simulink model "IEEE80211a"  (Simulink 10.0)
settings: Solver=VariableStepDiscrete  StartTime=0.0  StopTime=inf  RelTol=1e-3  EnableMultiTasking=on
PreLoadFcn:
  | load IEEE80211a_init;
undefined symbols (not defined in the file): hyst, j, magnitude, params, QAM, thres
libraries: simulink x27, IEEE80211a_lib x19, dspsigops x19, dspmtrx3 x19, dspsigattribs x15, dspmlti3 x10, dspstat3 x6, dspmathops x5, dspindex x3, dspsrcs4 x3, dspbuff3 x2, dspxfrm3 x2
(part 1 of 2)
CloseFcn:
  | IEEE80211a_open_graphics('IEEE80211a/MATLAB graphics', 1)
settings Model: Creator=Martin Clark  LastModifiedBy=bhisma
settings DataIOCC: LimitDataPoints=on  SignalLoggingSaveFormat=ModelDataLogs  SaveOutput=off  SaveTime=off  SignalLoggingName=sigsOut
settings OptimizationCC: LifeSpan=auto
settings DebuggingCC: SaveWithParameterizedLinksMsg=none  SignalResolutionControl=TryResolveAllWithWarning  MultiTaskDSMMsg=warning  MultiTaskCondExecSysMsg=none  SFUnexpectedBacktrackingDiag=error  SFNoUnconditionalDefaultTransitionDiag=error  SFExecutionAtInitializationDiag=warning  ArithmeticOperatorsInVariantConditions=error
settings HardwareCC: TargetUnknown=on
settings SFSimCC: SimUseLocalCustomCode=on  SimParseCustomCode=off  CustomCodeUndefinedFunction=FilterOut
settings RTWCC: RTWUseLocalCustomCode=on
settings CodeAppCC: StateflowObjectComments=off
settings GRTTargetCC: TargetLangStandard=C99 (ISO)

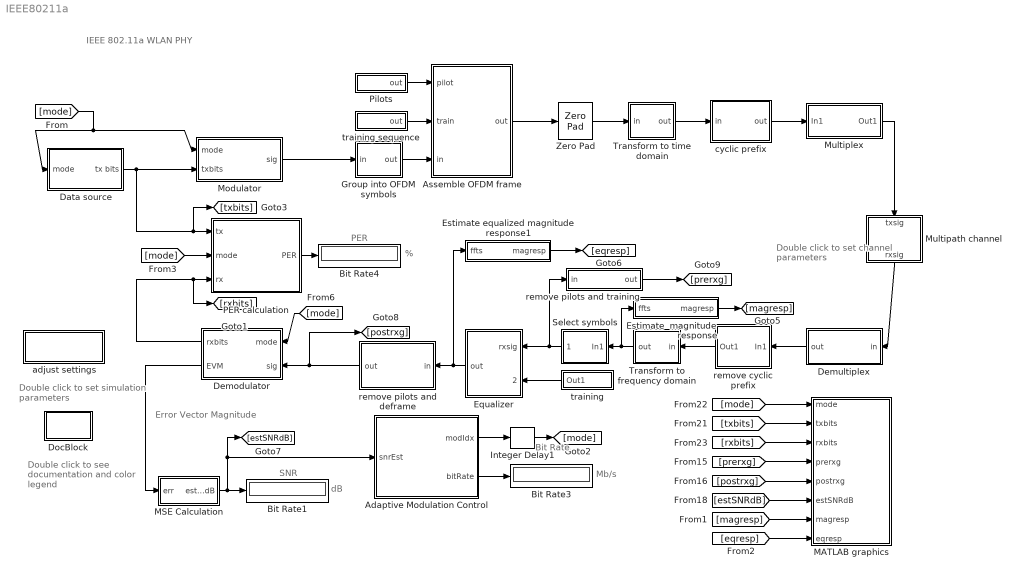
== system IEEE80211a ==
  note: IEEE 802.11a WLAN PHY
  note: Mb/s
  note: %
  note: Bit Rate
  note: Error Vector
      | Magnitude
  note: SNR
  note: dB
  note: Double click to set
      | channel parameters
  note: PER
  note: Double click to see
      |  documentation
      | and color legend
  note: Double click to set
      |  simulation parameters
  Adaptive Modulation Control : Stateflow chart  TreatAsAtomicUnit=on
  Assemble OFDM frame : Subsystem
      mask Display: disp('Assemble\nOFDM Frames')
  Bit Rate1 : Display
  Bit Rate3 : Display
  Bit Rate4 : Display
  Data source : Subsystem
      mask Display: disp('Variable-Rate\nData source')
  Demodulator : Subsystem  mask(IEEE 802.11a demodulator-decoder bank.){nSymbolsPerFrame=params.numTxSymbols, vtbd_set=params.vtbd_set}
      mask prompts: nSymbolsPerFrame "Number of symbols per frame:"; vtbd_set "vtbd set"
      mask init:
      | numModulators = 8;
      | modulation = {'BPSK' 'BPSK' 'QPSK' 'QPSK' '16-QAM' '16-QAM' '64-QAM' '64-QAM'};
      | code = {'1/2' '3/4' '1/2' '3/4' '1/2' '3/4' '2/3' '3/4'};
      | 
      | % modulation-specific
      | TS1 = 'poly2trellis(7, [171 133])';
      | TS2 = 'poly2trellis(7, [133 171])';
      | trellisStructure = {TS1 TS1 TS1 TS1 TS1 TS1 TS2 TS2};
      | 
      | % code-specific
      | PV = {'[1]', '[1 1 1 0].''', '[1 1 1 0 0 1].''', '[1]'};
      | punctureVector = {PV{1} PV{3} PV{1} PV{3} PV{1} PV{3} PV{2} PV{3}};
      | 
      | for n = 1:numModulators
      |     blk = [gcb '/Demodulator ' num2str(n)];
      |     set_param(blk, 'numSymbols', num2str(nSymbolsPerFrame));
      |     set_param(blk, 'modulation', modulation{n});
      |     set_param(blk, 'code', code{n});
      |     set_param(blk, 'trellisStructure', trellisStructure{n});
      |     set_param(blk, 'punctureVector', punctureVector{n});
      | end
      mask Display: disp('Demodulator\nBank')
  Demultiplex : Subsystem
      mask Display: disp('Demultiplex\nOFDM Frames')
  DocBlock : Subsystem  mask(DocBlock){ECoderFlag=, DocumentType=Text}
      mask prompts: ECoderFlag "E Coder Flag"; DocumentType "Document Type"
      mask help: Use this block to save long descriptive text with the model. Double-clicking the block will open an editor.
      settings: CopyFcn=docblock('breaklink',gcb);  DeleteFcn=docblock('close_document',gcb);  PreSaveFcn=docblock('save_document',gcb);  OpenFcn=docblock('edit_document',gcb);
      mask TypeOptions DocumentType: Text | RTF | HTML
      mask Display:
      | plot([.8 0 0 1 1 .8 .8 1],[1 1 0 0 .8 1 .8 .8]);
      | text(.5,.5,'DOC','horizontalalignment','center');
  Equalizer : Subsystem
      mask Display: disp('Frequency\nDomain\nEqualizer')
  Estimate  magnitude response : Subsystem
      mask Display: disp('Power Spectrum')
  Estimate equalized magnitude response1 : Subsystem
      mask Display: disp('Power Spectrum')
  Group into OFDM symbols : Subsystem
      mask Display: disp('OFDM\nSymbols')
  Integer Delay1 : dspsigops/Integer Delay  delay=1  ic=1  reset_popup=None
      settings: AttributesFormatString=\n  SourceProductName=DSP System Toolbox  SourceProductBaseCode=DS
  MATLAB graphics : Subsystem  mask(User-defined graphics.){graphicsName=IEEE80211a_graphics, portNames={'mode', 'txbits', 'rxbits', 'avSNRdB', 'prerxg', 'postrxg', 'estSNRdB', 'magresp', 'eqresp'}, convertMode=structure, extraParams=params}
      mask prompts: graphicsName "Graphics filename (without .fig or .m extension):"; portNames "Port names (cell array):"; convertMode "Data conversion mode:"; extraParams "Additional parameters:"
      mask init:
      | % derive input_names
      | bl = length(gcb);
      | long_names = find_system(gcb,...
      |     'lookundermasks','All',...
      |     'searchdepth', 1,...
      |     'BlockType','Inport');
      | lln = length(long_names);
      | input_names = cell(1, lln);
      | for i=1:lln
      | 	input_names{i}=long_names{i}(bl+2 : end);
      | end
      | 
      | if strcmp(get_param(gcb, 'LinkStatus'), 'resolved')
      | 	set_param(gcb, 'LinkStatus', 'inactive');
      | end
      settings: OpenFcn=IEEE80211a_open_graphics(gcb, 0);
      mask TypeOptions convertMode: cell array | structure
      mask Display: disp('Signal\nVisualization\n\nDouble click to\nopen/close')
  MSE Calculation : Subsystem
      mask Display: disp('SNR\nEstimation')
  Modulator : Subsystem  mask(IEEE 802.11a modulator-coder bank.){nSymbolsPerFrame=params.numTxSymbols}
      mask prompts: nSymbolsPerFrame "Number of symbols per frame:"
      mask init:
      | numModulators = 8;
      | modulation = {'BPSK' 'BPSK' 'QPSK' 'QPSK' '16-QAM' '16-QAM' '64-QAM' '64-QAM'};
      | code = {'1/2' '3/4' '1/2' '3/4' '1/2' '3/4' '2/3' '3/4'};
      | 
      | % modulation-specific
      | TS1 = 'poly2trellis(7, [171 133])';
      | TS2 = 'poly2trellis(7, [133 171])';
      | trellisStructure = {TS1 TS1 TS1 TS1 TS1 TS1 TS2 TS2};
      | 
      | % code-specific
      | PV = {'[1]', '[1 1 1 0].''', '[1 1 1 0 0 1].''', '[1]'};
      | punctureVector = {PV{1} PV{3} PV{1} PV{3} PV{1} PV{3} PV{2} PV{3}};
      | 
      | for n = 1:numModulators
      |     blk = [gcb '/Modulator ' num2str(n)];
      |     set_param(blk, 'numSymbols', num2str(nSymbolsPerFrame));
      |     set_param(blk, 'modulation', modulation{n});
      |     set_param(blk, 'code', code{n});
      |     set_param(blk, 'trellisStructure', trellisStructure{n});
      |     set_param(blk, 'punctureVector', punctureVector{n});
      | end
      mask Display: disp('Modulator\nBank')
  Multipath channel : Subsystem  mask(Multipath channel model parameters.){fadingMode=Dispersive fading, maxDoppler=200, SNRdB=30, chanSamplePeriod=params.chanSamplePeriod}
      mask prompts: fadingMode "Fading mode:"; maxDoppler "Maximum Doppler shift (Hz):"; SNRdB "SNR (dB):"; chanSamplePeriod "Channel sample period (s):"
      mask TypeOptions fadingMode: No fading | Flat fading | Dispersive fading
      mask Display: disp('Multipath\nChannel')
  Multiplex : Subsystem
      mask Display: disp('Multiplex\nOFDM Frames')
  PER calculation : Subsystem
      mask Display: disp('Packet Error Rate\nCalculation')
  Pilots : Subsystem
      mask Display: disp('Pilots')
  Select symbols : Subsystem
      mask Display: disp('Remove\nZeros')
  Transform to frequency domain : Subsystem
      mask Display: disp('FFT')
  Transform to time domain : Subsystem
      mask Display: disp('IFFT')
  Zero Pad : dspsigops/Zero Pad  padSigAt=End  zpadAlong=Columns  padNumOutRowsSpecMethod=User-specified  numOutRows=params.NFFT  padNumOutColsSpecMethod=User-specified  numOutCols=1  trunc_flag=None
      settings: SourceProductName=DSP System Toolbox  SourceProductBaseCode=DS
  adjust settings : Subsystem  Priority=1  mask(IEEE 802.11a model - Settings.){symbol_period=0.08e-6, OFDMSymPerFrame=20, OFDMTrainPerFrame=4, SNR0_dB=[10 11 14 18 22 26 28], hyst=3, vtbd=34}
      mask prompts: symbol_period "Symbol period (seconds):"; OFDMSymPerFrame "Number of OFDM symbols per transmit block:"; OFDMTrainPerFrame "Number of OFDM symbols in training sequence:"; SNR0_dB "Low-SNR thresholds (dB) -- no threshold for lowest modulation:"; hyst "Hysteresis factor for adaptive modulation (dB):"; vtbd "Viterbi traceback depth:"
      mask help: Parameter settings for IEEE 802.11a model.
      mask init:
      | params = IEEE80211a_settings(...
      | 	symbol_period, ...
      | 	OFDMSymPerFrame, ...
      | 	OFDMTrainPerFrame, ...
      | 	vtbd);
      | 
      | assignin('base', 'params', params);
      | assignin('base', 'thres', SNR0_dB);
      | assignin('base', 'hyst', hyst);
      mask Help: Parameter settings for IEEE 802.11a model.
      mask Display: disp('Simulation\nSettings')
  cyclic prefix : Subsystem
      mask Display: disp('Append\nCyclic\nPrefix')
  remove cyclic prefix : Subsystem
      mask Display: disp('Remove\nCyclic\nPrefix')
  remove pilots and deframe : Subsystem
      mask Display: disp('Disassemble\nOFDM Frames')
  remove pilots and training : Subsystem
      mask Display: disp('Constellation')
  training : Subsystem
      mask Display: disp('Training')
  training sequence : Subsystem
      mask Display: disp('Training')
  wires:
  cyclic prefix/1(out) -> Multiplex/1(In1)
  [mode] -> Demodulator/1(mode)
  Modulator/1(sig) -> Group into OFDM symbols/1(in)
  Demodulator/2(EVM) -> MSE Calculation/1(err)
  Data source/1(tx bits) -> Modulator/2(txbits), PER calculation/1(tx), [txbits]
  PER calculation/1(PER) -> Bit Rate4/1
  Demodulator/1(rxbits) -> PER calculation/3(rx), [rxbits]
  Integer Delay1/1 -> [mode]
  Adaptive Modulation Control/2(bitRate) -> Bit Rate3/1
  Adaptive Modulation Control/1(modIdx) -> Integer Delay1/1
  Transform to time domain/1(out) -> cyclic prefix/1(in)
  Assemble OFDM frame/1(out) -> Zero Pad/1
  training sequence/1(out) -> Assemble OFDM frame/2(train)
  Pilots/1(out) -> Assemble OFDM frame/1(pilot)
  Estimate  magnitude response/1(magresp) -> [magresp]
  Estimate equalized magnitude response1/1(magresp) -> [eqresp]
  Multipath channel/1(rxsig) -> Demultiplex/1(in)
  remove cyclic prefix/1(Out1) -> Transform to frequency domain/1(in)
  Equalizer/1(out) -> remove pilots and deframe/1(in), Estimate equalized magnitude response1/1(ffts)
  remove pilots and deframe/1(out) -> [postrxg], Demodulator/2(sig)
  training/1(Out1) -> Equalizer/2(trainsig)
  Transform to frequency domain/1(out) -> Estimate  magnitude response/1(ffts), Select symbols/1(In1)
  Group into OFDM symbols/1(out) -> Assemble OFDM frame/3(in)
  Multiplex/1(Out1) -> Multipath channel/1(txsig)
  Demultiplex/1(out) -> remove cyclic prefix/1(In1)
  [mode] -> Data source/1(mode), Modulator/1(mode)
  Zero Pad/1 -> Transform to time domain/1(in)
  remove pilots and training/1(out) -> [prerxg]
  Select symbols/1(Out1) -> Equalizer/1(rxsig), remove pilots and training/1(in)
  MSE Calculation/1(estSNRdB) -> Bit Rate1/1, Adaptive Modulation Control/1(snrEst), [estSNRdB]
  [mode] -> MATLAB graphics/1(mode)
  [txbits] -> MATLAB graphics/2(txbits)
  [rxbits] -> MATLAB graphics/3(rxbits)
  [prerxg] -> MATLAB graphics/4(prerxg)
  [postrxg] -> MATLAB graphics/5(postrxg)
  [estSNRdB] -> MATLAB graphics/6(estSNRdB)
  [magresp] -> MATLAB graphics/7(magresp)
  [eqresp] -> MATLAB graphics/8(eqresp)
  [mode] -> PER calculation/2(mode)

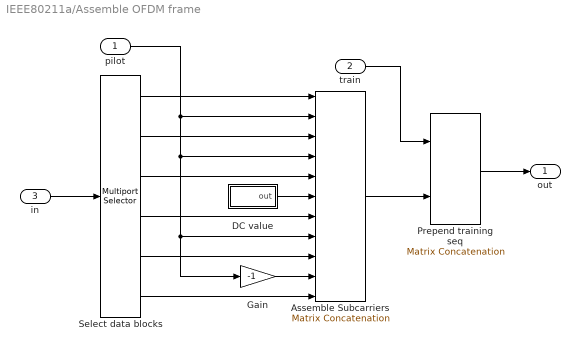
== system IEEE80211a/Assemble OFDM frame ==
  pilot : Inport
  train : Inport  Port=2
  in : Inport  Port=3
  Assemble Subcarriers : simulink/Math Operations/Matrix Concatenation  numInports=11  catMethod=Vertical
      settings: SourceProductName=Simulink  SourceProductBaseCode=SL
  DC value : Subsystem
      mask Display: disp('Zero DC')
  Gain : Gain  Gain=-1  SaturateOnIntegerOverflow=on  OutDataTypeStr=Inherit: Same as input  ParamDataTypeStr=Inherit: Same as input
  Prepend training seq : simulink/Math Operations/Matrix Concatenation  numInports=2  catMethod=Horizontal
      settings: SourceProductName=Simulink  SourceProductBaseCode=SL
  Select data blocks : dspindex/Multiport Selector  rowsOrCols=Rows  idxCellArray={1:5, 6:18, 19:24, 25:30, 31:43, 44:48}  idxErrMode=Clip Index
  out : Outport
  wires:
  Select data blocks/1 -> Assemble Subcarriers/1
  Select data blocks/2 -> Assemble Subcarriers/3
  Select data blocks/3 -> Assemble Subcarriers/5
  Select data blocks/4 -> Assemble Subcarriers/7
  Select data blocks/5 -> Assemble Subcarriers/9
  Select data blocks/6 -> Assemble Subcarriers/11
  Gain/1 -> Assemble Subcarriers/10
  pilot/1 -> Gain/1, Assemble Subcarriers/8, Assemble Subcarriers/4, Assemble Subcarriers/2
  Assemble Subcarriers/1 -> Prepend training seq/2
  train/1 -> Prepend training seq/1
  Prepend training seq/1 -> out/1
  DC value/1(out) -> Assemble Subcarriers/6
  in/1 -> Select data blocks/1

== system IEEE80211a/Data source ==
  mode : Inport
  Binary source : Subsystem  TreatAsAtomicUnit=on  mask{sample_time=params.minBitPeriod, samp_per_frame=params.nSource}
      mask prompts: sample_time "Sample time:"; samp_per_frame "Samples per frame:"
      mask help: Enabled binary data source
  Buffer : dspbuff3/Buffer  N=params.maxBitsPerBlock  V=0  ic=0
      settings: SourceProductName=DSP System Toolbox  SourceProductBaseCode=DS
  Source enable : Subsystem
  tx bits : Outport
  wires:
  Binary source/1(data out) -> Buffer/1
  Buffer/1 -> tx bits/1
  mode/1 -> Source enable/1(mode)
  Source enable/1(enable) -> Binary source/Enable

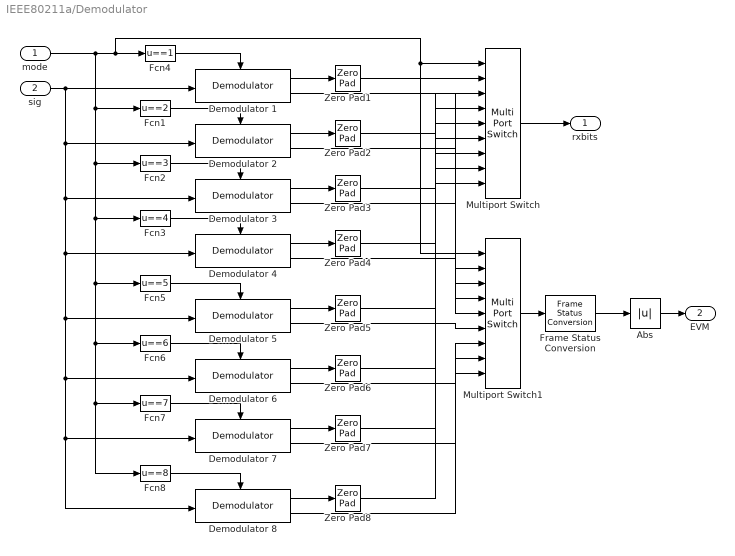
== system IEEE80211a/Demodulator ==
  mode : Inport
  sig : Inport  Port=2
  Abs : Abs  SaturateOnIntegerOverflow=on
  Demodulator 1 : IEEE80211a_lib/Demodulator  numSymbols=960  modulation=BPSK  code=1/2  trellisStructure=poly2trellis(7, [171 133])  punctureVector=[1]  vtbd=34
  Demodulator 2 : IEEE80211a_lib/Demodulator  numSymbols=960  modulation=BPSK  code=3/4  trellisStructure=poly2trellis(7, [171 133])  punctureVector=[1 1 1 0 0 1].'  vtbd=34
  Demodulator 3 : IEEE80211a_lib/Demodulator  numSymbols=960  modulation=QPSK  code=1/2  trellisStructure=poly2trellis(7, [171 133])  punctureVector=[1]  vtbd=34
  Demodulator 4 : IEEE80211a_lib/Demodulator  numSymbols=960  modulation=QPSK  code=3/4  trellisStructure=poly2trellis(7, [171 133])  punctureVector=[1 1 1 0 0 1].'  vtbd=34
  Demodulator 5 : IEEE80211a_lib/Demodulator  numSymbols=960  modulation=16-QAM  code=1/2  trellisStructure=poly2trellis(7, [171 133])  punctureVector=[1]  vtbd=34
  Demodulator 6 : IEEE80211a_lib/Demodulator  numSymbols=960  modulation=16-QAM  code=3/4  trellisStructure=poly2trellis(7, [171 133])  punctureVector=[1 1 1 0 0 1].'  vtbd=34
  Demodulator 7 : IEEE80211a_lib/Demodulator  numSymbols=960  modulation=64-QAM  code=2/3  trellisStructure=poly2trellis(7, [133 171])  punctureVector=[1 1 1 0].'  vtbd=34
  Demodulator 8 : IEEE80211a_lib/Demodulator  numSymbols=960  modulation=64-QAM  code=3/4  trellisStructure=poly2trellis(7, [133 171])  punctureVector=[1 1 1 0 0 1].'  vtbd=34
  Fcn1 : Fcn  Expr=u==2
  Fcn2 : Fcn  Expr=u==3
  Fcn3 : Fcn  Expr=u==4
  Fcn4 : Fcn  Expr=u==1
  Fcn5 : Fcn  Expr=u==5
  Fcn6 : Fcn  Expr=u==6
  Fcn7 : Fcn  Expr=u==7
  Fcn8 : Fcn  Expr=u==8
  Frame Status Conversion : dspsigattribs/Frame Status Conversion  growRefPort=off  outframe=Sample-based
      settings: SourceProductName=DSP System Toolbox  SourceProductBaseCode=DS
  Multiport Switch : MultiPortSwitch  Inputs=8  SaturateOnIntegerOverflow=on
  Multiport Switch1 : MultiPortSwitch  Inputs=8  SaturateOnIntegerOverflow=on
  Zero Pad{1..8} (8 alike) : dspsigops/Zero Pad  padSigAt=End  zpadAlong=Columns  padNumOutRowsSpecMethod=User-specified  numOutRows=4320  padNumOutColsSpecMethod=User-specified  numOutCols=1  trunc_flag=None
      settings: AttributesFormatString=\n  SourceProductName=DSP System Toolbox  SourceProductBaseCode=DS
  rxbits : Outport
  EVM : Outport  Port=2
  wires:
  sig/1 -> Demodulator 4/1, Demodulator 7/1, Demodulator 8/1, Demodulator 6/1, Demodulator 5/1, Demodulator 3/1, Demodulator 2/1, Demodulator 1/1
  mode/1 -> Fcn7/1, Fcn8/1, Fcn6/1, Fcn5/1, Fcn3/1, Fcn2/1, Fcn1/1, Multiport Switch/1, Multiport Switch1/1, Fcn4/1
  Multiport Switch/1 -> rxbits/1
  Zero Pad1/1 -> Multiport Switch/2
  Demodulator 8/1 -> Zero Pad8/1
  Demodulator 7/1 -> Zero Pad7/1
  Demodulator 6/1 -> Zero Pad6/1
  Demodulator 4/1 -> Zero Pad4/1
  Demodulator 5/1 -> Zero Pad5/1
  Demodulator 2/1 -> Zero Pad2/1
  Multiport Switch1/1 -> Frame Status Conversion/1
  Demodulator 1/2 -> Multiport Switch1/2
  Demodulator 2/2 -> Multiport Switch1/3
  Demodulator 3/2 -> Multiport Switch1/4
  Demodulator 5/2 -> Multiport Switch1/6
  Demodulator 6/2 -> Multiport Switch1/7
  Demodulator 7/2 -> Multiport Switch1/8
  Demodulator 8/2 -> Multiport Switch1/9
  Demodulator 4/2 -> Multiport Switch1/5
  Zero Pad2/1 -> Multiport Switch/3
  Zero Pad3/1 -> Multiport Switch/4
  Zero Pad4/1 -> Multiport Switch/5
  Zero Pad5/1 -> Multiport Switch/6
  Zero Pad6/1 -> Multiport Switch/7
  Zero Pad7/1 -> Multiport Switch/8
  Zero Pad8/1 -> Multiport Switch/9
  Fcn4/1 -> Demodulator 1/Enable
  Fcn1/1 -> Demodulator 2/Enable
  Fcn2/1 -> Demodulator 3/Enable
  Fcn3/1 -> Demodulator 4/Enable
  Fcn5/1 -> Demodulator 5/Enable
  Fcn6/1 -> Demodulator 6/Enable
  Fcn7/1 -> Demodulator 7/Enable
  Fcn8/1 -> Demodulator 8/Enable
  Demodulator 1/1 -> Zero Pad1/1
  Demodulator 3/1 -> Zero Pad3/1
  Frame Status Conversion/1 -> Abs/1
  Abs/1 -> EVM/1

== system IEEE80211a/Demultiplex ==
  in : Inport
  Demultiplex : simulink/Math Operations/Reshape  OutputDimensionality=Customize  OutputDimensions="[params.NFFT2  params.OFDMTotSymPerFrame]"
      settings: SourceProductName=Simulink  SourceProductBaseCode=SL
  out : Outport
  wires:
  Demultiplex/1 -> out/1
  in/1 -> Demultiplex/1

== system IEEE80211a/DocBlock ==
  EmptySubsystem : Subsystem

== system IEEE80211a/Equalizer ==
  note: data
  rxsig : Inport
  trainsig : Inport  Port=2
  Equalizer gains : Subsystem
  Product1 : Product  Inputs=/*  SaturateOnIntegerOverflow=on  OutDataTypeStr=Inherit: Same as first input
  Product2 : Product  Inputs=**  SaturateOnIntegerOverflow=on  OutDataTypeStr=Inherit: Same as first input
  Remove DC component : Selector  NumberOfDimensions=2  InputPortWidth=53  IndexOptions=Index vector (dialog),Select all  Indices=[1:26 28:53],-1  OutputSizes=1
  Remove training DC component : Selector  NumberOfDimensions=2  InputPortWidth=53  IndexOptions=Index vector (dialog),Select all  Indices=[1:26 28:53],-1  OutputSizes=1
  Select training/data : dspindex/Multiport Selector  rowsOrCols=Columns  idxCellArray={1:params.OFDMTrainPerFrame, params.OFDMTrainPerFrame+1:params.OFDMTotSymPerFrame}  idxErrMode=Clip Index
  out : Outport
  wires:
  rxsig/1 -> Remove DC component/1
  Select training/data/2 -> Product2/2
  Product2/1 -> out/1
  Equalizer gains/1(gains) -> Product2/1
  trainsig/1 -> Remove training DC component/1
  Product1/1 -> Equalizer gains/1(ch est)
  Select training/data/1 -> Product1/2
  Remove DC component/1 -> Select training/data/1
  Remove training DC component/1 -> Product1/1

== system IEEE80211a/Estimate  magnitude response ==
  ffts : Inport
  Math Function : Math  Operator=magnitude^2  SaturateOnIntegerOverflow=on
  Mean : dspstat3/Mean  run=off  reset_popup=None
  Transpose : dspmtrx3/Transpose  Hermitian=off
      settings: SourceProductName=DSP System Toolbox  SourceProductBaseCode=DS
  Transpose1 : dspmtrx3/Transpose  Hermitian=off
      settings: SourceProductName=DSP System Toolbox  SourceProductBaseCode=DS
  dB Conversion : dspmathops/dB Conversion  dBtype=dB  intype=Power  R=1  fuzz=on
      settings: SourceProductName=DSP System Toolbox
  magresp : Outport
  wires:
  dB Conversion/1 -> magresp/1
  Transpose1/1 -> dB Conversion/1
  Transpose/1 -> Mean/1
  Mean/1 -> Transpose1/1
  ffts/1 -> Math Function/1
  Math Function/1 -> Transpose/1

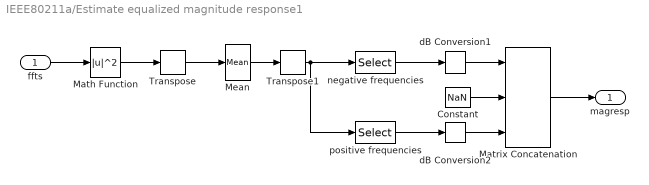
== system IEEE80211a/Estimate equalized magnitude response1 ==
  ffts : Inport
  Constant : Constant  Value=NaN
  Math Function : Math  Operator=magnitude^2  SaturateOnIntegerOverflow=on
  Matrix Concatenation : simulink/Math Operations/Matrix Concatenation  numInports=3  catMethod=Vertical
      settings: SourceProductName=Simulink  SourceProductBaseCode=SL
  Mean : dspstat3/Mean  run=off  reset_popup=None
  Transpose : dspmtrx3/Transpose  Hermitian=off
      settings: SourceProductName=DSP System Toolbox  SourceProductBaseCode=DS
  Transpose1 : dspmtrx3/Transpose  Hermitian=off
      settings: SourceProductName=DSP System Toolbox  SourceProductBaseCode=DS
  dB Conversion1 : dspmathops/dB Conversion  dBtype=dB  intype=Power  R=1  fuzz=on
      settings: SourceProductName=DSP System Toolbox
  dB Conversion2 : dspmathops/dB Conversion  dBtype=dB  intype=Power  R=1  fuzz=on
      settings: SourceProductName=DSP System Toolbox
  negative frequencies : Selector  InputPortWidth=params.NST  IndexOptions=Index vector (dialog)  Indices=[1:params.NST/2]  OutputSizes=1
  positive frequencies : Selector  InputPortWidth=params.NST  IndexOptions=Index vector (dialog)  Indices=params.NST/2+1:params.NST  OutputSizes=1
  magresp : Outport
  wires:
  Constant/1 -> Matrix Concatenation/2
  Matrix Concatenation/1 -> magresp/1
  dB Conversion2/1 -> Matrix Concatenation/3
  positive frequencies/1 -> dB Conversion2/1
  dB Conversion1/1 -> Matrix Concatenation/1
  negative frequencies/1 -> dB Conversion1/1
  Transpose1/1 -> positive frequencies/1, negative frequencies/1
  Transpose/1 -> Mean/1
  Mean/1 -> Transpose1/1
  ffts/1 -> Math Function/1
  Math Function/1 -> Transpose/1

== system IEEE80211a/Group into OFDM symbols ==
  in : Inport
  "Group data for OFDM symbols " : simulink/Math Operations/Reshape  OutputDimensionality=Customize  OutputDimensions=[params.NSD params.OFDMSymPerFrame]
      settings: SourceProductName=Simulink  SourceProductBaseCode=SL
  out : Outport
  wires:
  in/1 -> "Group data for OFDM symbols "/1
  "Group data for OFDM symbols "/1 -> out/1

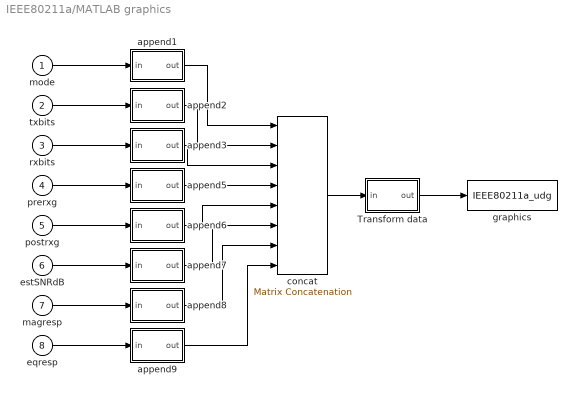
== system IEEE80211a/MATLAB graphics ==
  mode : Inport
  txbits : Inport  Port=2
  rxbits : Inport  Port=3
  prerxg : Inport  Port=4
  postrxg : Inport  Port=5
  estSNRdB : Inport  Port=6
  magresp : Inport  Port=7
  eqresp : Inport  Port=8
  Transform data : Subsystem
      mask Display: disp('Transform\nData')
  append1 : Subsystem
      mask Display: disp('Append\nSize')
  append2 : Subsystem
      mask Display: disp('Append\nSize')
  append3 : Subsystem
      mask Display: disp('Append\nSize')
  append5 : Subsystem
      mask Display: disp('Append\nSize')
  append6 : Subsystem
      mask Display: disp('Append\nSize')
  append7 : Subsystem
      mask Display: disp('Append\nSize')
  append8 : Subsystem
      mask Display: disp('Append\nSize')
  append9 : Subsystem
      mask Display: disp('Append\nSize')
  concat : simulink/Math Operations/Matrix Concatenation  numInports=8  catMethod=Vertical
      settings: SourceProductName=Simulink  SourceProductBaseCode=SL
  graphics : S-Function  FunctionName=IEEE80211a_udg  Parameters={input_names, extraParams}  SFunctionDeploymentMode=off  EnableBusSupport=off
  wires:
  eqresp/1 -> append9/1(in)
  magresp/1 -> append8/1(in)
  estSNRdB/1 -> append7/1(in)
  postrxg/1 -> append6/1(in)
  prerxg/1 -> append5/1(in)
  rxbits/1 -> append3/1(in)
  txbits/1 -> append2/1(in)
  Transform data/1(out) -> graphics/1
  concat/1 -> Transform data/1(in)
  mode/1 -> append1/1(in)
  append1/1(out) -> concat/1
  append2/1(out) -> concat/2
  append3/1(out) -> concat/3
  append9/1(out) -> concat/8
  append8/1(out) -> concat/7
  append7/1(out) -> concat/6
  append6/1(out) -> concat/5
  append5/1(out) -> concat/4

== system IEEE80211a/MSE Calculation ==
  err : Inport
  Math Function2 : Math  Operator=reciprocal  SaturateOnIntegerOverflow=on
  Matrix Square : dspmtrx3/Matrix Square
      settings: SourceProductName=DSP System Toolbox  SourceProductBaseCode=DS
  RMS : dspstat3/RMS  run=off  reset_popup=None
  dB Conversion : dspmathops/dB Conversion  dBtype=dB  intype=Power  R=1  fuzz=on
      settings: SourceProductName=DSP System Toolbox
  estSNRdB : Outport
  wires:
  Matrix Square/1 -> Math Function2/1
  Math Function2/1 -> dB Conversion/1
  RMS/1 -> Matrix Square/1
  err/1 -> RMS/1
  dB Conversion/1 -> estSNRdB/1

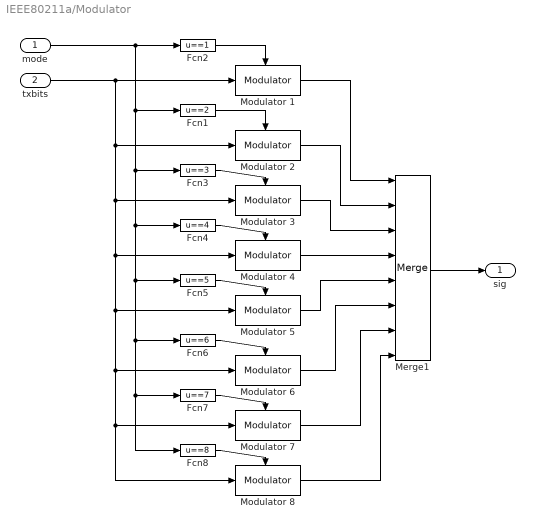
== system IEEE80211a/Modulator ==
  mode : Inport
  txbits : Inport  Port=2
  Fcn1 : Fcn  Expr=u==2
  Fcn2 : Fcn  Expr=u==1
  Fcn3 : Fcn  Expr=u==3
  Fcn4 : Fcn  Expr=u==4
  Fcn5 : Fcn  Expr=u==5
  Fcn6 : Fcn  Expr=u==6
  Fcn7 : Fcn  Expr=u==7
  Fcn8 : Fcn  Expr=u==8
  Merge1 : Merge  Inputs=8
  Modulator 1 : IEEE80211a_lib/Modulator  numSymbols=960  modulation=BPSK  code=1/2  trellisStructure=poly2trellis(7, [171 133])  punctureVector=[1]
  Modulator 2 : IEEE80211a_lib/Modulator  numSymbols=960  modulation=BPSK  code=3/4  trellisStructure=poly2trellis(7, [171 133])  punctureVector=[1 1 1 0 0 1].'
  Modulator 3 : IEEE80211a_lib/Modulator  numSymbols=960  modulation=QPSK  code=1/2  trellisStructure=poly2trellis(7, [171 133])  punctureVector=[1]
  Modulator 4 : IEEE80211a_lib/Modulator  numSymbols=960  modulation=QPSK  code=3/4  trellisStructure=poly2trellis(7, [171 133])  punctureVector=[1 1 1 0 0 1].'
  Modulator 5 : IEEE80211a_lib/Modulator  numSymbols=960  modulation=16-QAM  code=1/2  trellisStructure=poly2trellis(7, [171 133])  punctureVector=[1]
  Modulator 6 : IEEE80211a_lib/Modulator  numSymbols=960  modulation=16-QAM  code=3/4  trellisStructure=poly2trellis(7, [171 133])  punctureVector=[1 1 1 0 0 1].'
  Modulator 7 : IEEE80211a_lib/Modulator  numSymbols=960  modulation=64-QAM  code=2/3  trellisStructure=poly2trellis(7, [133 171])  punctureVector=[1 1 1 0].'
  Modulator 8 : IEEE80211a_lib/Modulator  numSymbols=960  modulation=64-QAM  code=3/4  trellisStructure=poly2trellis(7, [133 171])  punctureVector=[1 1 1 0 0 1].'
  sig : Outport
  wires:
  Merge1/1 -> sig/1
  mode/1 -> Fcn7/1, Fcn8/1, Fcn6/1, Fcn5/1, Fcn4/1, Fcn3/1, Fcn1/1, Fcn2/1
  txbits/1 -> Modulator 7/1, Modulator 8/1, Modulator 6/1, Modulator 5/1, Modulator 4/1, Modulator 3/1, Modulator 2/1, Modulator 1/1
  Modulator 1/1 -> Merge1/1
  Modulator 2/1 -> Merge1/2
  Modulator 3/1 -> Merge1/3
  Modulator 4/1 -> Merge1/4
  Modulator 5/1 -> Merge1/5
  Modulator 6/1 -> Merge1/6
  Modulator 7/1 -> Merge1/7
  Modulator 8/1 -> Merge1/8
  Fcn2/1 -> Modulator 1/Enable
  Fcn1/1 -> Modulator 2/Enable
  Fcn3/1 -> Modulator 3/Enable
  Fcn4/1 -> Modulator 4/Enable
  Fcn5/1 -> Modulator 5/Enable
  Fcn6/1 -> Modulator 6/Enable
  Fcn7/1 -> Modulator 7/Enable
  Fcn8/1 -> Modulator 8/Enable

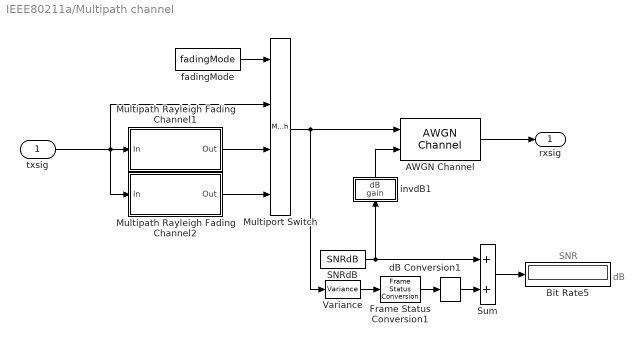
== system IEEE80211a/Multipath channel ==
  note: SNR
  note: dB
  txsig : Inport
  AWGN Channel : commchan2/AWGN Channel  seed=67  noiseMode=Variance from port  EsNodB=15  SNRdB=10  Ps=1  Tsym=1e-6  variance=1
      settings: SourceProductName=Communications Toolbox  SourceProductBaseCode=CM
  Bit Rate5 : Display
  Frame Status Conversion1 : dspsigattribs/Frame Status Conversion  growRefPort=off  outframe=Sample-based
      settings: SourceProductName=DSP System Toolbox  SourceProductBaseCode=DS
  Multipath Rayleigh Fading Channel1 : Subsystem  mask(Multipath Rayleigh Fading Channel){Fd=maxDoppler, simTs=chanSamplePeriod, delayVec=0, gainVecdB=0, normGain=on, Seed=73}
      mask prompts: Fd "Maximum Doppler shift (Hz):"; simTs "Sample time:"; delayVec "Delay vector (s):"; gainVecdB "Gain vector (dB):"; normGain "Normalize gain vector to 0 dB overall gain"; Seed "Initial seed:"
      mask help:
      | Multipath Rayleigh fading channel for complex baseband signals.
      |
      | Multiplies the input signal with samples of a Rayleigh distributed complex random process. The spectrum of the Rayleigh process is given by the Jakes PSD.
      |
      | The number of paths equals the length of either the 'Delay vector' or 'Gain vector' parameters.
      mask init:
      | commblkrayleighchan2(gcb);
      mask Help: helpview(commbhelp)
      mask Display:
      | plot(0,0,100,100,[05 15 10 10 05 10 18 14 13 7.5 13 41 44 47 50 53 57 59 100-[13 7.5 13 14 18 10 5 10 10 15 5]],[70 70 70 85 92 85 79 82 90 88.5 90 90 87 93 87 93 87 90 90 88.5 90 82 79 85 92 85 70 70 70]);
      | disp('Multipath\nRayleigh Fading')
  Multipath Rayleigh Fading Channel2 : Subsystem  mask(Multipath Rayleigh Fading Channel){Fd=maxDoppler, simTs=chanSamplePeriod, delayVec=[0 chanSamplePeriod], gainVecdB=[0 -3], normGain=on, Seed=73}
      mask prompts: Fd "Maximum Doppler shift (Hz):"; simTs "Sample time:"; delayVec "Delay vector (s):"; gainVecdB "Gain vector (dB):"; normGain "Normalize gain vector to 0 dB overall gain"; Seed "Initial seed:"
      mask help:
      | Multipath Rayleigh fading channel for complex baseband signals.
      |
      | Multiplies the input signal with samples of a Rayleigh distributed complex random process. The spectrum of the Rayleigh process is given by the Jakes PSD.
      |
      | The number of paths equals the length of either the 'Delay vector' or 'Gain vector' parameters.
      mask init:
      | commblkrayleighchan2(gcb);
      mask Help: helpview(commbhelp)
      mask Display:
      | plot(0,0,100,100,[05 15 10 10 05 10 18 14 13 7.5 13 41 44 47 50 53 57 59 100-[13 7.5 13 14 18 10 5 10 10 15 5]],[70 70 70 85 92 85 79 82 90 88.5 90 90 87 93 87 93 87 90 90 88.5 90 82 79 85 92 85 70 70 70]);
      | disp('Multipath\nRayleigh Fading')
  Multiport Switch : MultiPortSwitch  SaturateOnIntegerOverflow=on
  SNRdB : Constant  Value=SNRdB
  Sum : Sum  SaturateOnIntegerOverflow=on
  Variance : dspstat3/Variance  run=off  reset_popup=None
      settings: SourceProductName=DSP System Toolbox
  dB Conversion1 : dspmathops/dB Conversion  dBtype=dB  intype=Power  R=1  fuzz=on
      settings: SourceProductName=DSP System Toolbox
  fadingMode : Constant  Value=fadingMode
  invdB1 : Subsystem
      mask Display: disp('1/invdB')
  rxsig : Outport
  wires:
  SNRdB/1 -> invdB1/1(gain), Sum/1
  txsig/1 -> Multipath Rayleigh Fading Channel1/1(In), Multiport Switch/2, Multipath Rayleigh Fading Channel2/1(In)
  AWGN Channel/1 -> rxsig/1
  Multiport Switch/1 -> AWGN Channel/1, Variance/1
  Multipath Rayleigh Fading Channel1/1(Out) -> Multiport Switch/3
  Multipath Rayleigh Fading Channel2/1(Out) -> Multiport Switch/4
  fadingMode/1 -> Multiport Switch/1
  Sum/1 -> Bit Rate5/1
  invdB1/1(dB) -> AWGN Channel/2
  Frame Status Conversion1/1 -> dB Conversion1/1
  Variance/1 -> Frame Status Conversion1/1
  dB Conversion1/1 -> Sum/2

== system IEEE80211a/Multiplex ==
  In1 : Inport
  Reshape2 : simulink/Math Operations/Reshape  OutputDimensionality=Column vector  OutputDimensions=1600
      settings: SourceProductName=Simulink  SourceProductBaseCode=SL
  Out1 : Outport
  wires:
  In1/1 -> Reshape2/1
  Reshape2/1 -> Out1/1

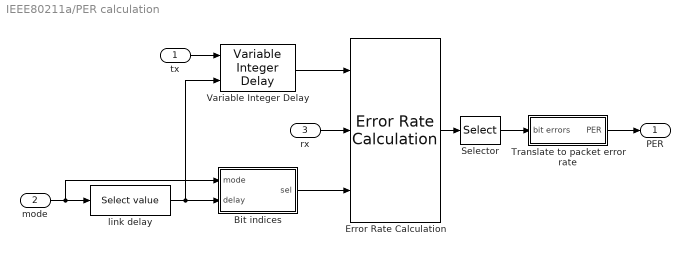
== system IEEE80211a/PER calculation ==
  tx : Inport
  mode : Inport  Port=2
  rx : Inport  Port=3
  Bit indices : Subsystem
  Error Rate Calculation : commsink2/Error Rate Calculation  N=0  st_delay=0  cp_mode=Select samples from port  subframe=[]  PMode=Port  WsName=ErrorVec  RsMode2=off  stop=off  numErr=100  maxBits=1e6
      settings: SourceProductName=Communications Toolbox
  Selector : Selector  InputPortWidth=3  IndexOptions=Index vector (dialog)  Indices=2  OutputSizes=1
  Translate to packet error rate : Subsystem
  Variable Integer Delay : dspsigops/Variable Integer Delay  dmax=100  ic=0
      settings: SourceProductName=DSP System Toolbox  SourceProductBaseCode=DS
  link delay : IEEE80211a_lib/Select value  vector=params.link_delay.'
  PER : Outport
  wires:
  rx/1 -> Error Rate Calculation/2
  link delay/1 -> Bit indices/2(delay), Variable Integer Delay/2
  Selector/1 -> Translate to packet error rate/1(bit errors)
  Translate to packet error rate/1(PER) -> PER/1
  Variable Integer Delay/1 -> Error Rate Calculation/1
  Bit indices/1(sel) -> Error Rate Calculation/3
  mode/1 -> Bit indices/1(mode), link delay/1
  Error Rate Calculation/1 -> Selector/1
  tx/1 -> Variable Integer Delay/1

== system IEEE80211a/Pilots ==
  PN Sequence Generator : commseqgen2/PN Sequence Generator  poly=[1 0 0 0 1 0 0 1]  ini_sta=[1 1 1 1 1 1 1]  shift=0  Ts=params.blockPeriod/params.OFDMSymPerFrame  frameBased=on  sampPerFrame=params.OFDMSymPerFrame  reset=off
      settings: SourceProductName=Communications Toolbox  SourceProductBaseCode=CM
  Reshape : simulink/Math Operations/Reshape  OutputDimensionality=Row vector  OutputDimensions=[1,1]
      settings: SourceProductName=Simulink  SourceProductBaseCode=SL
  Unipolar to Bipolar Converter : commutil2/Unipolar to Bipolar Converter  M=2  polarity=Negative
      settings: SourceProductName=Communications Toolbox
  out : Outport
  wires:
  Reshape/1 -> out/1
  Unipolar to Bipolar Converter/1 -> Reshape/1
  PN Sequence Generator/1 -> Unipolar to Bipolar Converter/1

== system IEEE80211a/Select symbols ==
  In1 : Inport
  Select symbols : Selector  NumberOfDimensions=2  InputPortWidth=64  IndexOptions=Index vector (dialog),Select all  Indices=params.RXSelectFFTIndices,-1  OutputSizes=1
  Out1 : Outport
  wires:
  In1/1 -> Select symbols/1
  Select symbols/1 -> Out1/1

== system IEEE80211a/Transform to frequency domain ==
  in : Inport
  FFT : dspxfrm3/FFT  CompMethod=Table lookup  TableOpt=Speed  BitRevOrder=off
  Frame Status Conversion : dspsigattribs/Frame Status Conversion  growRefPort=off  outframe=Frame-based
      settings: SourceProductName=DSP System Toolbox  SourceProductBaseCode=DS
  Normalize : Gain  Gain=1/sqrt(params.NFFT)/(sqrt(params.NFFT/params.NST))  SaturateOnIntegerOverflow=on  OutDataTypeStr=Inherit: Same as input  ParamDataTypeStr=Inherit: Same as input
  out : Outport
  wires:
  FFT/1 -> Normalize/1
  Normalize/1 -> Frame Status Conversion/1
  in/1 -> FFT/1
  Frame Status Conversion/1 -> out/1

== system IEEE80211a/Transform to time domain ==
  in : Inport
  IFFT : dspxfrm3/IFFT  CompMethod=Table lookup  TableOpt=Speed  BitRevOrder=off  cs_in=off  SkipNorm=off  mode=Complex
      settings: SourceProductName=DSP System Toolbox
  Normalize : Gain  Gain=sqrt(params.NFFT)*sqrt(params.NFFT/params.NST)  SaturateOnIntegerOverflow=on  OutDataTypeStr=Inherit: Same as input  ParamDataTypeStr=Inherit: Same as input
  Shift for FFT : Selector  NumberOfDimensions=2  InputPortWidth=64  IndexOptions=Index vector (dialog),Select all  Indices=params.TXFFTShiftIndices,-1  OutputSizes=1
  out : Outport
  wires:
  Shift for FFT/1 -> IFFT/1
  in/1 -> Shift for FFT/1
  IFFT/1 -> Normalize/1
  Normalize/1 -> out/1

== system IEEE80211a/adjust settings ==
  note: This subsystem is empty.
      | It is used for setting parameter values (in the mask).

== system IEEE80211a/cyclic prefix ==
  in : Inport
  Add Cyclic Prefix : Selector  NumberOfDimensions=2  InputPortWidth=64  IndexOptions=Index vector (dialog),Select all  Indices=params.TXCyclicPrefixIndices,-1  OutputSizes=1
  out : Outport
  wires:
  Add Cyclic Prefix/1 -> out/1
  in/1 -> Add Cyclic Prefix/1

== system IEEE80211a/remove cyclic prefix ==
  In1 : Inport
  Remove cyclic prefix : Selector  NumberOfDimensions=2  InputPortWidth=80  IndexOptions=Index vector (dialog),Select all  Indices=params.RXCyclicPrefixIndices,-1  OutputSizes=1
  Out1 : Outport
  wires:
  In1/1 -> Remove cyclic prefix/1
  Remove cyclic prefix/1 -> Out1/1

== system IEEE80211a/remove pilots and deframe ==
  in : Inport
  Remove pilots : dspindex/Multiport Selector  rowsOrCols=Rows  idxCellArray={[1:5 7:19 21:32 34:46 48:52], [6 20 33 47]}  idxErrMode=Clip Index
  Reshape3 : simulink/Math Operations/Reshape  OutputDimensionality=Column vector  OutputDimensions=960
      settings: SourceProductName=Simulink  SourceProductBaseCode=SL
  Terminator : Terminator
  out : Outport
  wires:
  Remove pilots/2 -> Terminator/1  "Pilots"
  Remove pilots/1 -> Reshape3/1  "Data"
  Reshape3/1 -> out/1
  in/1 -> Remove pilots/1

== system IEEE80211a/remove pilots and training ==
  in : Inport
  Frame Status Conversion : dspsigattribs/Frame Status Conversion  growRefPort=off  outframe=Sample-based
      settings: SourceProductName=DSP System Toolbox  SourceProductBaseCode=DS
  Remove DC component : Selector  NumberOfDimensions=2  InputPortWidth=53  IndexOptions=Index vector (dialog),Select all  Indices=[1:26 28:53],-1  OutputSizes=1
  Remove training and pilots : Selector  NumberOfDimensions=2  InputPortWidth=80  IndexOptions=Index vector (dialog),Index vector (dialog)  Indices=[1:5 7:19 21:32 34:46 48:52],params.OFDMTrainPerFrame+1:params.OFDMTotSymPerFrame  OutputSizes=1
  Reshape5 : simulink/Math Operations/Reshape  OutputDimensionality=Column vector  OutputDimensions=960
      settings: SourceProductName=Simulink  SourceProductBaseCode=SL
  out : Outport
  wires:
  Remove training and pilots/1 -> Reshape5/1
  Remove DC component/1 -> Remove training and pilots/1
  in/1 -> Remove DC component/1
  Reshape5/1 -> Frame Status Conversion/1
  Frame Status Conversion/1 -> out/1

== system IEEE80211a/training ==
  Frame Status Conversion : dspsigattribs/Frame Status Conversion  growRefPort=off  outframe=Frame-based
      settings: SourceProductName=DSP System Toolbox  SourceProductBaseCode=DS
  Training sequence : Constant  Value=repmat(params.long_training_seq, [1 params.OFDMTrainPerFrame])
  Out1 : Outport
  wires:
  Training sequence/1 -> Frame Status Conversion/1
  Frame Status Conversion/1 -> Out1/1

== system IEEE80211a/training sequence ==
  Frame Status Conversion : dspsigattribs/Frame Status Conversion  growRefPort=off  outframe=Frame-based
      settings: SourceProductName=DSP System Toolbox  SourceProductBaseCode=DS
  Training sequence : Constant  Value=repmat(params.long_training_seq, [1 params.OFDMTrainPerFrame])
  out : Outport
  wires:
  Training sequence/1 -> Frame Status Conversion/1
  Frame Status Conversion/1 -> out/1

== system IEEE80211a/Assemble OFDM frame/DC value ==
  Constant : Constant  Value=complex(zeros(1,params.OFDMSymPerFrame))  VectorParams1D=off
  Frame Status Conversion : dspsigattribs/Frame Status Conversion  growRefPort=off  outframe=Frame-based
      settings: SourceProductName=DSP System Toolbox  SourceProductBaseCode=DS
  out : Outport
  wires:
  Constant/1 -> Frame Status Conversion/1
  Frame Status Conversion/1 -> out/1

== system IEEE80211a/Data source/Binary source ==
  Enable : EnablePort
  Constant : Constant  Value=0.5
  Random Source : dspsrcs4/Random Source  SrcType=Uniform  NormMethod=Ziggurat  CltLength=12  Min=0  Max=1  Mean=0  Var=1  RepMode=Specify seed  Seed=61  Inherit=off  SampMode=Discrete  SampTime=sample_time  SampFrame=samp_per_frame  DataType=Double  OutComplex=Real
  Relational Operator : RelationalOperator  Operator=>  OutDataTypeStr=float('double')  RndMeth=Nearest  InputSameDT=on
  data out : Outport  OutputWhenDisabled=reset  InitialOutput=0
  wires:
  Random Source/1 -> Relational Operator/1
  Constant/1 -> Relational Operator/2
  Relational Operator/1 -> data out/1

== system IEEE80211a/Data source/Source enable ==
  mode : Inport
  Constant : Constant  Value=(1:max(params.nS)).'
  Relational Operator1 : RelationalOperator  Operator=<=  OutDataTypeStr=float('double')  RndMeth=Nearest  InputSameDT=on
  Unbuffer : dspbuff3/Unbuffer  ic=0
      settings: SourceProductName=DSP System Toolbox  SourceProductBaseCode=DS
  slot size : IEEE80211a_lib/Select value  vector=params.nS.'
  enable : Outport
  wires:
  slot size/1 -> Relational Operator1/2
  Constant/1 -> Relational Operator1/1
  Relational Operator1/1 -> Unbuffer/1
  Unbuffer/1 -> enable/1
  mode/1 -> slot size/1

== system IEEE80211a/DocBlock/EmptySubsystem ==

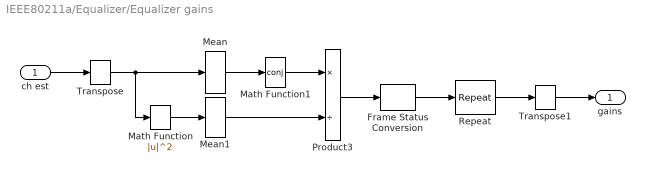
== system IEEE80211a/Equalizer/Equalizer gains ==
  ch est : Inport
  Frame Status Conversion : dspsigattribs/Frame Status Conversion  growRefPort=off  outframe=Frame-based
      settings: SourceProductName=DSP System Toolbox  SourceProductBaseCode=DS
  Math Function : Math  Operator=magnitude^2  SaturateOnIntegerOverflow=on
  Math Function1 : Math  Operator=conj  SaturateOnIntegerOverflow=on
  Mean : dspstat3/Mean  run=off  reset_popup=None
  Mean1 : dspstat3/Mean  run=off  reset_popup=None
  Product3 : Product  Inputs=*/  SaturateOnIntegerOverflow=on  OutDataTypeStr=Inherit: Same as first input
  Repeat : dspsigops/Repeat  N=params.OFDMSymPerFrame  ic=0  mode=Maintain input frame rate
      settings: SourceProductName=DSP System Toolbox
  Transpose : dspmtrx3/Transpose  Hermitian=off
      settings: SourceProductName=DSP System Toolbox  SourceProductBaseCode=DS
  Transpose1 : dspmtrx3/Transpose  Hermitian=off
      settings: SourceProductName=DSP System Toolbox  SourceProductBaseCode=DS
  gains : Outport
  wires:
  ch est/1 -> Transpose/1
  Math Function/1 -> Mean1/1
  Mean/1 -> Math Function1/1
  Mean1/1 -> Product3/2
  Math Function1/1 -> Product3/1
  Product3/1 -> Frame Status Conversion/1
  Transpose/1 -> Math Function/1, Mean/1
  Frame Status Conversion/1 -> Repeat/1
  Repeat/1 -> Transpose1/1
  Transpose1/1 -> gains/1

== system IEEE80211a/MATLAB graphics/Transform data ==
  in : Inport
  Complex to Real-Imag : ComplexToRealImag
  Concatenate : simulink/Math Operations/Matrix Concatenation  numInports=2  catMethod=Horizontal
      settings: SourceProductName=Simulink  SourceProductBaseCode=SL
  Frame Status Conversion : dspsigattribs/Frame Status Conversion  growRefPort=off  outframe=Sample-based
      settings: SourceProductName=DSP System Toolbox  SourceProductBaseCode=DS
  out : Outport
  wires:
  Frame Status Conversion/1 -> out/1
  in/1 -> Complex to Real-Imag/1
  Complex to Real-Imag/1 -> Concatenate/1
  Complex to Real-Imag/2 -> Concatenate/2
  Concatenate/1 -> Frame Status Conversion/1

== system IEEE80211a/MATLAB graphics/append1 ==
  in : Inport
  Matrix Concatenation1 : simulink/Math Operations/Matrix Concatenation  numInports=2  catMethod=Vertical
      settings: SourceProductName=Simulink  SourceProductBaseCode=SL
  Reshape : simulink/Math Operations/Reshape  OutputDimensionality=Column vector  OutputDimensions=[1,1]
      settings: SourceProductName=Simulink  SourceProductBaseCode=SL
  Transpose : dspmtrx3/Transpose  Hermitian=off
      settings: AttributesFormatString=\n  SourceProductName=DSP System Toolbox  SourceProductBaseCode=DS
  Width : Width
  out : Outport
  wires:
  in/1 -> Width/1, Reshape/1
  Width/1 -> Transpose/1
  Reshape/1 -> Matrix Concatenation1/2
  Transpose/1 -> Matrix Concatenation1/1
  Matrix Concatenation1/1 -> out/1

== system IEEE80211a/MATLAB graphics/append2 ==
  in : Inport
  Matrix Concatenation1 : simulink/Math Operations/Matrix Concatenation  numInports=2  catMethod=Vertical
      settings: SourceProductName=Simulink  SourceProductBaseCode=SL
  Reshape : simulink/Math Operations/Reshape  OutputDimensionality=Column vector  OutputDimensions=[1,1]
      settings: SourceProductName=Simulink  SourceProductBaseCode=SL
  Transpose : dspmtrx3/Transpose  Hermitian=off
      settings: AttributesFormatString=\n  SourceProductName=DSP System Toolbox  SourceProductBaseCode=DS
  Width : Width
  out : Outport
  wires:
  Matrix Concatenation1/1 -> out/1
  Transpose/1 -> Matrix Concatenation1/1
  Reshape/1 -> Matrix Concatenation1/2
  Width/1 -> Transpose/1
  in/1 -> Reshape/1, Width/1

== system IEEE80211a/MATLAB graphics/append3 ==
  in : Inport
  Matrix Concatenation1 : simulink/Math Operations/Matrix Concatenation  numInports=2  catMethod=Vertical
      settings: SourceProductName=Simulink  SourceProductBaseCode=SL
  Reshape : simulink/Math Operations/Reshape  OutputDimensionality=Column vector  OutputDimensions=[1,1]
      settings: SourceProductName=Simulink  SourceProductBaseCode=SL
  Transpose : dspmtrx3/Transpose  Hermitian=off
      settings: AttributesFormatString=\n  SourceProductName=DSP System Toolbox  SourceProductBaseCode=DS
  Width : Width
  out : Outport
  wires:
  Matrix Concatenation1/1 -> out/1
  Transpose/1 -> Matrix Concatenation1/1
  Reshape/1 -> Matrix Concatenation1/2
  Width/1 -> Transpose/1
  in/1 -> Reshape/1, Width/1

== system IEEE80211a/MATLAB graphics/append5 ==
  in : Inport
  Matrix Concatenation1 : simulink/Math Operations/Matrix Concatenation  numInports=2  catMethod=Vertical
      settings: SourceProductName=Simulink  SourceProductBaseCode=SL
  Reshape : simulink/Math Operations/Reshape  OutputDimensionality=Column vector  OutputDimensions=[1,1]
      settings: SourceProductName=Simulink  SourceProductBaseCode=SL
  Transpose : dspmtrx3/Transpose  Hermitian=off
      settings: AttributesFormatString=\n  SourceProductName=DSP System Toolbox  SourceProductBaseCode=DS
  Width : Width
  out : Outport
  wires:
  Matrix Concatenation1/1 -> out/1
  Transpose/1 -> Matrix Concatenation1/1
  Reshape/1 -> Matrix Concatenation1/2
  Width/1 -> Transpose/1
  in/1 -> Reshape/1, Width/1

== system IEEE80211a/MATLAB graphics/append6 ==
  in : Inport
  Matrix Concatenation1 : simulink/Math Operations/Matrix Concatenation  numInports=2  catMethod=Vertical
      settings: SourceProductName=Simulink  SourceProductBaseCode=SL
  Reshape : simulink/Math Operations/Reshape  OutputDimensionality=Column vector  OutputDimensions=[1,1]
      settings: SourceProductName=Simulink  SourceProductBaseCode=SL
  Transpose : dspmtrx3/Transpose  Hermitian=off
      settings: AttributesFormatString=\n  SourceProductName=DSP System Toolbox  SourceProductBaseCode=DS
  Width : Width
  out : Outport
  wires:
  Matrix Concatenation1/1 -> out/1
  Transpose/1 -> Matrix Concatenation1/1
  Reshape/1 -> Matrix Concatenation1/2
  Width/1 -> Transpose/1
  in/1 -> Reshape/1, Width/1

== system IEEE80211a/MATLAB graphics/append7 ==
  in : Inport
  Matrix Concatenation1 : simulink/Math Operations/Matrix Concatenation  numInports=2  catMethod=Vertical
      settings: SourceProductName=Simulink  SourceProductBaseCode=SL
  Reshape : simulink/Math Operations/Reshape  OutputDimensionality=Column vector  OutputDimensions=[1,1]
      settings: SourceProductName=Simulink  SourceProductBaseCode=SL
  Transpose : dspmtrx3/Transpose  Hermitian=off
      settings: AttributesFormatString=\n  SourceProductName=DSP System Toolbox  SourceProductBaseCode=DS
  Width : Width
  out : Outport
  wires:
  Matrix Concatenation1/1 -> out/1
  Transpose/1 -> Matrix Concatenation1/1
  Reshape/1 -> Matrix Concatenation1/2
  Width/1 -> Transpose/1
  in/1 -> Reshape/1, Width/1

== system IEEE80211a/MATLAB graphics/append8 ==
  in : Inport
  Matrix Concatenation1 : simulink/Math Operations/Matrix Concatenation  numInports=2  catMethod=Vertical
      settings: SourceProductName=Simulink  SourceProductBaseCode=SL
  Reshape : simulink/Math Operations/Reshape  OutputDimensionality=Column vector  OutputDimensions=[1,1]
      settings: SourceProductName=Simulink  SourceProductBaseCode=SL
  Transpose : dspmtrx3/Transpose  Hermitian=off
      settings: AttributesFormatString=\n  SourceProductName=DSP System Toolbox  SourceProductBaseCode=DS
  Width : Width
  out : Outport
  wires:
  Matrix Concatenation1/1 -> out/1
  Transpose/1 -> Matrix Concatenation1/1
  Reshape/1 -> Matrix Concatenation1/2
  Width/1 -> Transpose/1
  in/1 -> Reshape/1, Width/1

== system IEEE80211a/MATLAB graphics/append9 ==
  in : Inport
  Matrix Concatenation1 : simulink/Math Operations/Matrix Concatenation  numInports=2  catMethod=Vertical
      settings: SourceProductName=Simulink  SourceProductBaseCode=SL
  Reshape : simulink/Math Operations/Reshape  OutputDimensionality=Column vector  OutputDimensions=[1,1]
      settings: SourceProductName=Simulink  SourceProductBaseCode=SL
  Transpose : dspmtrx3/Transpose  Hermitian=off
      settings: AttributesFormatString=\n  SourceProductName=DSP System Toolbox  SourceProductBaseCode=DS
  Width : Width
  out : Outport
  wires:
  Matrix Concatenation1/1 -> out/1
  Transpose/1 -> Matrix Concatenation1/1
  Reshape/1 -> Matrix Concatenation1/2
  Width/1 -> Transpose/1
  in/1 -> Reshape/1, Width/1

== system IEEE80211a/Multipath channel/Multipath Rayleigh Fading Channel1 ==
  In : Inport
  Multipath Fading Channel : Subsystem  mask(Multipath Fading Channel){Fd=Fd, LOSFd=0, K=0, simTs=simTs, delayVec=delayVec, gainVecdB=gainVecdB, normGain=on, Seed=Seed}
      mask prompts: Fd "Doppler frequency (Hz):"; LOSFd "Line-of-sight Doppler frequency (Hz):"; K "K-factor:"; simTs "Sample time (sec):"; delayVec "Delay vector (sec):"; gainVecdB "Gain vector (dB):"; normGain "Normalize gain vector to 0 dB overall gain"; Seed "Initial seed:"
      mask help:
      | Multipath fading channel for complex baseband signals.
      |
      | Multiplies the input signal with samples of a complex random process. The spectrum of the random process is given by the Jakes PSD, where the Doppler frequency parameter determines the maximum Doppler frequency. The K-factor parameter specifies the linear ratio of power in the direct path to the diffuse power.
      |
      | The number of paths equals the length of either the 'Delay vector' or 'Gain vector' parameters.
      mask init:
      | [ecode,emsg,params] = commblkfadingchan2(gcb,Fd,LOSFd,K,simTs,delayVec,gainVecdB,normGain,Seed);
      | if(ecode==1)
      |     error(emsg);
      | elseif(ecode==2)
      |     warning(emsg);
      | end;
      mask Display:
      | plot(0,0,100,100,[05 15 10 10 05 10 18 14 13 7.5 13 41 44 47 50 53 57 59 100-[13 7.5 13 14 18 10 5 10 10 15 5]],[70 70 70 85 92 85 79 82 90 88.5 90 90 87 93 87 93 87 90 90 88.5 90 82 79 85 92 85 70 70 70]);
      | disp('Multipath\nFading')
  Out : Outport
  wires:
  Multipath Fading Channel/1(Out) -> Out/1
  In/1 -> Multipath Fading Channel/1(In)
